simulink library "Energy_converter_Electrical_to_Mechanical"  (R2016a)
settings: Solver=ode1  StartTime=0.0  StopTime=Inf  FixedStep=0.001  RelTol=1e-3
undefined symbols (not defined in the file): API1dcac_efficiency, API2dcac_efficiency, API3dcac_efficiency, aux_power_state, AWR_InvStError, dat, DiscIntNeverNeededParam, EDCU_p_RefTqeMOT, emot_AcCmprFront_inertia, emot_AcCmprFront_nTab_3rdD, emot_AcCmprFront_pwrAC, emot_AcCmprFront_Tau, emot_AcCmprFront_trqTab_2ndD, emot_AcCmprFront_vltTab_1stD, emot_AcCmprRear_inertia, emot_AcCmprRear_nTab_3rdD, emot_AcCmprRear_pwrAC, emot_AcCmprRear_Tau, emot_AcCmprRear_trqTab_2ndD, emot_AcCmprRear_vltTab_1stD, emot_AirCmpr_inertia, emot_AirCmpr_nTab_3rdD, emot_AirCmpr_pwrAC, emot_AirCmpr_Tau, emot_AirCmpr_trqTab_2ndD, emot_AirCmpr_vltTab_1stD, emot_aircomp_power, emot_Cth_rotor, emot_Cth_stator, emot_dtrqEmotNeg, emot_dtrqEmotPtv, emot_inv_pwracTab_1st, emot_inv_pwrDC, emot_inv_pwrLoss, emot_inv_VrmsTab_2nd, emot_j, emot_mot_pwrLoss, emot_nTab_1stD, emot_pwrEtaTab_nRow, emot_pwrEtaTab_pwrTab, emot_pwrEtaTab_trqClm, emot_Rth_rotor_oil, emot_Rth_stator_oil, emot_Rth_stator_rotor, emot_tractiongroup, emot_Trotor_init, emot_trqMaxRow, emot_trqMinRow, emot_Tstator_init, emot_vltTab_3rdD, FirstDrivenAxleNoOfEmot, inv_Cth_cooling_plate, inv_Cth_diode, inv_Cth_IGBT, inv_n_IGBT_per_Switch, inv_Rth_cooling_plate_coolant, inv_Rth_PS_cooling_plate, inv_Tplate_init, inv_Tpowerstack_init, midAxleNoOfEmot ... (+6)
libraries: Electrical_converter x12, Energy_converter_Electrical_to_Mechanical x12, simulink x7
(part 3 of 8)

== system Energy_converter_Electrical_to_Mechanical/Emot AC Compressor Front ==
  hvs_emot_AcCompressorFront_torque : Inport
  hvs_DcLink_voltage_API1 : Inport  Port=2
  hvsAux_InverterAcCompressorFront_torque_Rq : Inport  Port=3
  hvsaux_EmotAcCompressorFront_Voltage_Rq : Inport  Port=4
  Avoid_Div_by_zero : Subsystem
  Constant1 : Constant  Value=0
  Constant2 : Constant  Value=0
  Constant5 : Constant  Value=emot_AcCmprFront_inertia
  Discrete Filter : DiscreteFilter  Numerator=[emot_AcCmprFront_Tau emot_AcCmprFront_Tau]  Denominator=[0.1+emot_AcCmprFront_Tau emot_AcCmprFront_Tau-0.1]
  Discrete-Time Integrator : DiscreteIntegrator  SampleTime=-1  ICPrevOutput=DiscIntNeverNeededParam  ICPrevScaledInput=DiscIntNeverNeededParam
  Gain1 : Gain
      settings: AttributesFormatString=%<Description>
  Gain2 : Gain  SampleTime=K
      mask init:
      | K = str2num(get_param(bdroot,'FixedStep'));
  Gain3 : Gain  Gain=30/pi
      settings: AttributesFormatString=%<Description>
  Product1 : Product  Inputs=*/  RndMeth=Zero
  Product2 : Product  Inputs=**  RndMeth=Zero
  Rate Transition : RateTransition
  Rate Transition1 : RateTransition
  Saturation : Saturate  UpperLimit=Inf  LowerLimit=0
  Subtract : Sum  Inputs=+-
  Subtract1 : Sum  Inputs=+-
  Switch : Switch  Criteria=u2 > Threshold
  W_to_kW : Gain  Gain=1/1000
      settings: AttributesFormatString=%<Description>
  efficiency : Gain  Gain=1/API3dcac_efficiency
      settings: AttributesFormatString=%<Description>
  motor mode : Lookup_n-D  NumberOfTableDimensions=3  BreakpointsForDimension1=emot_AcCmprFront_vltTab_1stD  BreakpointsForDimension2=emot_AcCmprFront_trqTab_2ndD  BreakpointsForDimension3=emot_AcCmprFront_nTab_3rdD  Table=emot_AcCmprFront_pwrAC  ExtrapMethod=Clip  UseLastTableValue=on  InputSameDT=on
  hvs_emot_AirCondFrontHV_angAcc : Outport
  hvs_emot_AirCondFrontHV_angPos : Outport  Port=2
  hvs_emot_AirCondFrontHV_angVel : Outport  Port=3
  hvs_inverterAcCompressor_wasteHeat_power : Outport  Port=4
  hvs_InverterAcCompressorFront_hvCurrent : Outport  Port=5
  hvs_InverterAcCompressorFront_hvVoltage : Outport  Port=6
  hvs_emot_AcCompressorFront_nEmot : Outport  Port=7
  wires:
  W_to_kW/1 -> hvs_inverterAcCompressor_wasteHeat_power/1
  Gain2/1 -> Switch/2, motor mode/2, Subtract/1
  Subtract1/1 -> W_to_kW/1
  efficiency/1 -> Product2/1, Subtract1/1
  Switch/1 -> efficiency/1, Subtract1/2  "phys_current_A"
  Product2/1 -> hvs_InverterAcCompressorFront_hvCurrent/1
  Avoid_Div_by_zero/1(1/U) -> Product2/2
  hvs_DcLink_voltage_API1/1 -> Gain1/1, Avoid_Div_by_zero/1(U)
  Gain1/1 -> hvs_InverterAcCompressorFront_hvVoltage/1
  Constant1/1 -> Switch/3
  Constant2/1 -> hvs_emot_AirCondFrontHV_angPos/1
  hvsAux_InverterAcCompressorFront_torque_Rq/1 -> Discrete Filter/1
  hvsaux_EmotAcCompressorFront_Voltage_Rq/1 -> motor mode/1
  motor mode/1 -> Switch/1  "ElecMac_ElecPwr_W"
  Discrete Filter/1 -> Gain2/1
  hvs_emot_AcCompressorFront_torque/1 -> Subtract/2
  Subtract/1 -> Product1/1
  Constant5/1 -> Product1/2  "phys_inertia_kgm2"
  Product1/1 -> hvs_emot_AirCondFrontHV_angAcc/1, Rate Transition/1
  Discrete-Time Integrator/1 -> Saturation/1
  Saturation/1 -> hvs_emot_AirCondFrontHV_angVel/1, Gain3/1
  Rate Transition/1 -> Discrete-Time Integrator/1
  [angVel] -> Rate Transition1/1
  Rate Transition1/1 -> motor mode/3
  Gain3/1 -> hvs_emot_AcCompressorFront_nEmot/1, [angVel]

== system Energy_converter_Electrical_to_Mechanical/Emot AC Compressor Rear ==
  hvs_emot_AcCompressorRear_torque : Inport
  hvs_DcLink_voltage_API3 : Inport  Port=2
  hvsAux_InverterAcCompressorRear_torque_Rq : Inport  Port=3
  hvsaux_EmotAcCompressorRear_Voltage_Rq : Inport  Port=4
  Avoid_Div_by_zero : Subsystem
  Constant1 : Constant  Value=0
  Constant2 : Constant  Value=0
  Constant5 : Constant  Value=emot_AcCmprRear_inertia
  Discrete Filter : DiscreteFilter  Numerator=[emot_AcCmprRear_Tau emot_AcCmprRear_Tau]  Denominator=[0.1+emot_AcCmprRear_Tau emot_AcCmprRear_Tau-0.1]
  Discrete-Time Integrator : DiscreteIntegrator  SampleTime=-1  ICPrevOutput=DiscIntNeverNeededParam  ICPrevScaledInput=DiscIntNeverNeededParam
  Gain1 : Gain
      settings: AttributesFormatString=%<Description>
  Gain2 : Gain  SampleTime=K
      mask init:
      | K = str2num(get_param(bdroot,'FixedStep'));
  Gain3 : Gain  Gain=30/pi
      settings: AttributesFormatString=%<Description>
  Product1 : Product  Inputs=*/  RndMeth=Zero
  Product2 : Product  Inputs=**  RndMeth=Zero
  Rate Transition1 : RateTransition
  Rate Transition2 : RateTransition
  Saturation : Saturate  UpperLimit=Inf  LowerLimit=0
  Subtract : Sum  Inputs=+-
  Subtract1 : Sum  Inputs=+-
  Switch : Switch  Criteria=u2 > Threshold
  W_to_kW : Gain  Gain=1/1000
      settings: AttributesFormatString=%<Description>
  efficiency : Gain  Gain=1/API1dcac_efficiency
      settings: AttributesFormatString=%<Description>
  motor mode : Lookup_n-D  NumberOfTableDimensions=3  BreakpointsForDimension1=emot_AcCmprRear_vltTab_1stD  BreakpointsForDimension2=emot_AcCmprRear_trqTab_2ndD  BreakpointsForDimension3=emot_AcCmprRear_nTab_3rdD  Table=emot_AcCmprRear_pwrAC  ExtrapMethod=Clip  UseLastTableValue=on  InputSameDT=on
  hvs_emot_AirCondRearHV_angAcc : Outport
  hvs_emot_AirCondRearHV_angPos : Outport  Port=2
  hvs_emot_AirCondRearHV_angVel : Outport  Port=3
  hvs_inverterAcCompressorRear_wasteHeat_power : Outport  Port=4
  hvs_InverterAcCompressorRear_hvCurrent : Outport  Port=5
  hvs_InverterAcCompressorRear_hvVoltage : Outport  Port=6
  hvs_InverterAcCompressorRear_nEmot : Outport  Port=7
  wires:
  W_to_kW/1 -> hvs_inverterAcCompressorRear_wasteHeat_power/1
  Gain2/1 -> Subtract/1, Switch/2, motor mode/2
  Subtract1/1 -> W_to_kW/1
  efficiency/1 -> Subtract1/1, Product2/1
  Switch/1 -> efficiency/1, Subtract1/2  "phys_current_A"
  Avoid_Div_by_zero/1(1/U) -> Product2/2
  Product2/1 -> hvs_InverterAcCompressorRear_hvCurrent/1
  Gain1/1 -> hvs_InverterAcCompressorRear_hvVoltage/1
  hvs_DcLink_voltage_API3/1 -> Gain1/1, Avoid_Div_by_zero/1(U)
  Constant1/1 -> Switch/3
  Saturation/1 -> hvs_emot_AirCondRearHV_angVel/1, Gain3/1
  Discrete-Time Integrator/1 -> Saturation/1
  Product1/1 -> Rate Transition1/1, hvs_emot_AirCondRearHV_angAcc/1
  Constant5/1 -> Product1/2  "phys_inertia_kgm2"
  Subtract/1 -> Product1/1
  hvs_emot_AcCompressorRear_torque/1 -> Subtract/2
  Discrete Filter/1 -> Gain2/1
  motor mode/1 -> Switch/1  "ElecMac_ElecPwr_W"
  hvsaux_EmotAcCompressorRear_Voltage_Rq/1 -> motor mode/1
  hvsAux_InverterAcCompressorRear_torque_Rq/1 -> Discrete Filter/1
  Constant2/1 -> hvs_emot_AirCondRearHV_angPos/1
  Rate Transition1/1 -> Discrete-Time Integrator/1
  [angVel] -> Rate Transition2/1
  Rate Transition2/1 -> motor mode/3
  Gain3/1 -> [angVel], hvs_InverterAcCompressorRear_nEmot/1

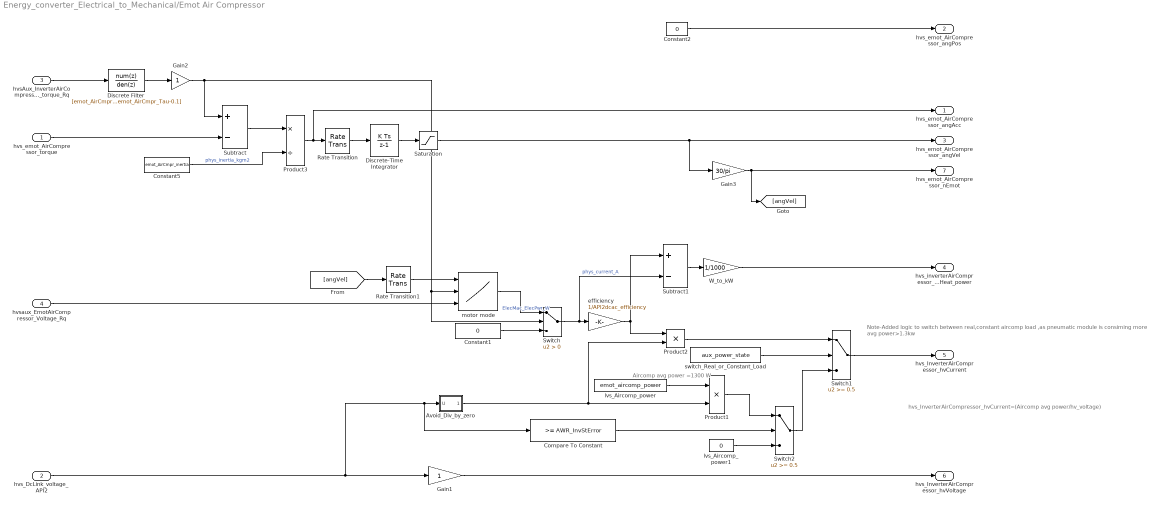
== system Energy_converter_Electrical_to_Mechanical/Emot Air Compressor ==
  note: Note-Added logic to switch between real,constant aircomp load ,as pneumatic module is consiming more avg power>1.3kw
  note: hvs_InverterAirCompressor_hvCurrent=(Aircomp avg power/hv_voltage)
  note: Aircomp avg power =1300 W
  hvs_emot_AirCompressor_torque : Inport
  hvs_DcLink_voltage_API2 : Inport  Port=2
  hvsAux_InverterAirCompressor_torque_Rq : Inport  Port=3
  hvsaux_EmotAirCompressor_Voltage_Rq : Inport  Port=4
  Avoid_Div_by_zero : Subsystem
  Compare To Constant : simulink/Logic and Bit Operations/Compare To Constant  relop=>=  const=AWR_InvStError  OutDataTypeStr=boolean
  Constant1 : Constant  Value=0
  Constant2 : Constant  Value=0
  Constant5 : Constant  Value=emot_AirCmpr_inertia
  Discrete Filter : DiscreteFilter  Numerator=[emot_AirCmpr_Tau emot_AirCmpr_Tau]  Denominator=[0.1+emot_AirCmpr_Tau emot_AirCmpr_Tau-0.1]
  Discrete-Time Integrator : DiscreteIntegrator  SampleTime=-1  ICPrevOutput=DiscIntNeverNeededParam  ICPrevScaledInput=DiscIntNeverNeededParam
  Gain1 : Gain
      settings: AttributesFormatString=%<Description>
  Gain2 : Gain  SampleTime=K
      mask init:
      | K = str2num(get_param(bdroot,'FixedStep'));
  Gain3 : Gain  Gain=30/pi
      settings: AttributesFormatString=%<Description>
  Product1 : Product  Inputs=**  RndMeth=Zero
  Product2 : Product  Inputs=**  RndMeth=Zero
  Product3 : Product  Inputs=*/  RndMeth=Zero
  Rate Transition : RateTransition
  Rate Transition1 : RateTransition
  Saturation : Saturate  UpperLimit=inf  LowerLimit=0
  Subtract : Sum  Inputs=+-
  Subtract1 : Sum  Inputs=+-
  Switch : Switch  Criteria=u2 > Threshold
  Switch1 : Switch  Threshold=0.5
  Switch2 : Switch  Threshold=0.5
  W_to_kW : Gain  Gain=1/1000
      settings: AttributesFormatString=%<Description>
  efficiency : Gain  Gain=1/API2dcac_efficiency
      settings: AttributesFormatString=%<Description>
  lvs_Aircomp_power : Constant  Value=emot_aircomp_power
  lvs_Aircomp_power1 : Constant  Value=0
  motor mode : Lookup_n-D  NumberOfTableDimensions=3  BreakpointsForDimension1=emot_AirCmpr_nTab_3rdD  BreakpointsForDimension2=emot_AirCmpr_trqTab_2ndD  BreakpointsForDimension3=emot_AirCmpr_vltTab_1stD  Table=emot_AirCmpr_pwrAC  ExtrapMethod=Clip  UseLastTableValue=on  InputSameDT=on
  switch_Real_or_Constant_Load : Constant  Value=aux_power_state
  hvs_emot_AirCompressor_angAcc : Outport
  hvs_emot_AirCompressor_angPos : Outport  Port=2
  hvs_emot_AirCompressor_angVel : Outport  Port=3
  hvs_inverterAirCompressor_wasteHeat_power : Outport  Port=4
  hvs_InverterAirCompressor_hvCurrent : Outport  Port=5
  hvs_InverterAirCompressor_hvVoltage : Outport  Port=6
  hvs_emot_AirCompressor_nEmot : Outport  Port=7
  wires:
  Switch2/1 -> Switch1/3
  Product1/1 -> Switch2/1
  Compare To Constant/1 -> Switch2/2
  lvs_Aircomp_power/1 -> Product1/1
  lvs_Aircomp_power1/1 -> Switch2/3
  hvs_DcLink_voltage_API2/1 -> Gain1/1, Avoid_Div_by_zero/1(U), Compare To Constant/1
  switch_Real_or_Constant_Load/1 -> Switch1/2
  Product2/1 -> Switch1/1
  Gain3/1 -> hvs_emot_AirCompressor_nEmot/1, [angVel]
  W_to_kW/1 -> hvs_inverterAirCompressor_wasteHeat_power/1
  Gain2/1 -> Subtract/1, Switch/2, motor mode/2
  Subtract1/1 -> W_to_kW/1
  efficiency/1 -> Product2/1, Subtract1/1
  Constant1/1 -> Switch/3
  Avoid_Div_by_zero/1(1/U) -> Product1/2, Product2/2
  Switch/1 -> efficiency/1, Subtract1/2  "phys_current_A"
  Gain1/1 -> hvs_InverterAirCompressor_hvVoltage/1
  hvsaux_EmotAirCompressor_Voltage_Rq/1 -> motor mode/3
  Saturation/1 -> hvs_emot_AirCompressor_angVel/1, Gain3/1
  Discrete-Time Integrator/1 -> Saturation/1
  Product3/1 -> Rate Transition/1, hvs_emot_AirCompressor_angAcc/1
  Constant5/1 -> Product3/2  "phys_inertia_kgm2"
  Subtract/1 -> Product3/1
  hvs_emot_AirCompressor_torque/1 -> Subtract/2
  Discrete Filter/1 -> Gain2/1
  motor mode/1 -> Switch/1  "ElecMac_ElecPwr_W"
  hvsAux_InverterAirCompressor_torque_Rq/1 -> Discrete Filter/1
  Constant2/1 -> hvs_emot_AirCompressor_angPos/1
  Rate Transition/1 -> Discrete-Time Integrator/1
  [angVel] -> Rate Transition1/1
  Rate Transition1/1 -> motor mode/1
  Switch1/1 -> hvs_InverterAirCompressor_hvCurrent/1

== system Energy_converter_Electrical_to_Mechanical/GTR_Electric_machine ==
  ElecMac_nReq_radps : Inport
  ElecMac_flgReqSwitch_B : Inport  Port=2
  ElecMac_tqReq_Nm : Inport  Port=3
  ElecMac_flowActCooling_kgps : Inport  Port=4
  el in [V] : Inport  Port=5
  mech fb in [rad/s] : Inport  Port=6
  Bus Creator : BusCreator  Inputs=2
  Bus Creator1 : BusCreator  Inputs=1
  Bus Creator2 : BusCreator  Inputs=5
  Bus Selector1 : BusSelector  OutputSignals=phys_voltage_V
  Bus Selector2 : BusSelector  OutputSignals=phys_speed_radps
  Bus Selector3 : BusSelector  OutputSignals=torque,ElecMac_flowActCooling_kgps
  Constant1 : Constant  Value=dat.inertia.value
  Gain{1..3,6} (4 alike) : Gain
  Product : Product  Inputs=/*  RndMeth=Zero
  Product1 : Product  Inputs=**  RndMeth=Zero
  Sum : Sum  Inputs=+-
  Switch : Switch
  Thermal : Subsystem
  Transfer Fcn1 : TransferFcn  Denominator=[dat.timeconstant.value 1]
  generator mode : Lookup_n-D  NumberOfTableDimensions=3  BreakpointsForDimension1=dat.elecpowmap.generator.voltage.vec  BreakpointsForDimension2=dat.elecpowmap.generator.torque.vec  BreakpointsForDimension3=dat.elecpowmap.generator.speed.vec  Table=dat.elecpowmap.generator.elecpow.map  ExtrapMethod=Clip  UseLastTableValue=on  InputSameDT=on
  local controller : Subsystem
  motor mode : Lookup_n-D  NumberOfTableDimensions=3  BreakpointsForDimension1=dat.elecpowmap.motor.voltage.vec  BreakpointsForDimension2=dat.elecpowmap.motor.torque.vec  BreakpointsForDimension3=dat.elecpowmap.motor.speed.vec  Table=dat.elecpowmap.motor.elecpow.map  ExtrapMethod=Clip  UseLastTableValue=on  InputSameDT=on
  mech out [Nm] : Outport
  el fb out [A] : Outport  Port=2
  Electric_speed_radps : Outport  Port=3
  wires:
  Sum/1 -> Thermal/1(Total power loss)
  Product1/1 -> Sum/2
  Thermal/1(Machine temperature[K]) -> Bus Creator2/4  "ElecMac_tAct_K"
  Gain6/1 -> Bus Creator/1  "phys_torque_Nm"
  Gain2/1 -> Bus Creator2/1  "ElecMac_tqAct_Nm"
  Gain1/1 -> Bus Creator2/2  "ElecMac_nAct_radps"
  Gain3/1 -> Bus Creator2/3  "ElecMac_iAct_A"
  Product/1 -> Gain3/1, Bus Creator1/1  "phys_current_A"
  Bus Selector3/1 -> Transfer Fcn1/1  "<torque>"
  Constant1/1 -> Bus Creator/2  "phys_inertia_kgm2"
  Bus Creator2/1 -> local controller/5(sensor in)
  Bus Selector2/1 -> Gain1/1, Product1/2, generator mode/3, motor mode/3  "<phys_speed_radps>"
  local controller/2(ctrl out) -> Bus Selector3/1
  mech fb in [rad/s]/1 -> Bus Selector2/1
  el in [V]/1 -> Bus Selector1/1
  Bus Creator/1 -> mech out [Nm]/1
  Bus Creator1/1 -> el fb out [A]/1
  motor mode/1 -> Switch/1  "ElecMac_ElecPwr_W"
  generator mode/1 -> Switch/3
  Switch/1 -> Product/2, Sum/1
  Bus Selector1/1 -> Product/1, motor mode/1, generator mode/1  "<phys_voltage_V>"
  Transfer Fcn1/1 -> Gain2/1, Gain6/1, Product1/1, generator mode/2, Switch/2, motor mode/2
  Bus Selector3/2 -> Thermal/2(Massflow cooling fluid)  "<ElecMac_flowActCooling_kgps>"
  Thermal/2(Fluid outlet temperature[K]) -> Bus Creator2/5  "ElecMac_tActCoolingOut_K"
  local controller/1(Electric_speed_radps) -> Electric_speed_radps/1
  ElecMac_nReq_radps/1 -> local controller/1(ElecMac_nReq_radps)
  ElecMac_flgReqSwitch_B/1 -> local controller/2(ElecMac_flgReqSwitch_B)
  ElecMac_tqReq_Nm/1 -> local controller/3(ElecMac_tqReq_Nm)
  ElecMac_flowActCooling_kgps/1 -> local controller/4(ElecMac_flowActCooling_kgps)

== system Energy_converter_Electrical_to_Mechanical/e-Motor ==
  nGbxEMIn : Inport
  voltBatHV : Inport  Port=2
  trqEmotDesPhy : Inport  Port=3
  emot_CMD : Inport  Port=4
  drvEmotOil_Temperature : Inport  Port=5
  drvInverter_Coolant_Temperature : Inport  Port=6
  Enable : EnablePort
  Constant2 : Constant  Value=0
  Fahrmotoren : Subsystem
  Gain : Gain  Gain=0.4
  Gain1 : Gain  Gain=0.6
  Switch : Switch  Threshold=0.5
  Thermic_Model_Inverter : Subsystem
  Thermic_Model_PMSM_slot2 : Subsystem
  Umrichter mit trq-Regler : Subsystem
  Unit Delay : UnitDelay  SampleTime=-1
  Unit Delay1 : UnitDelay  InitialCondition=emot_Tstator_init  SampleTime=-1
  Unit Delay2 : UnitDelay  InitialCondition=emot_Trotor_init  SampleTime=-1
  Unit Delay4 : UnitDelay  InitialCondition=inv_Tpowerstack_init  SampleTime=-1
  Unit Delay5 : UnitDelay  InitialCondition=inv_Tplate_init  SampleTime=-1
  updatePortNames : Subsystem
      settings: OpenFcn=std_PortNameFromSignal('Depth',2);
      mask Display: disp('updatePortNames')
  pwrEmotPhy : Outport
  Inv_Ploss : Outport  Port=2
  mot_Ploss : Outport  Port=3
  trqEmotPhy : Outport  Port=4
  trqEmotMax : Outport  Port=5
  drvEmot_wasteHeat_power : Outport  Port=6
  drvEmot_T_Stator : Outport  Port=7
  driveInverter_wasteHeat_power : Outport  Port=8
  driveInverter_T_Coolplate : Outport  Port=9
  wires:
  Thermic_Model_PMSM_slot2/3(T_Rotor_new) -> Unit Delay1/1  "drvEmot_T_Rotor"
  Unit Delay1/1 -> Thermic_Model_PMSM_slot2/5(T_Rotor)
  Thermic_Model_PMSM_slot2/2(T_Stator_new) -> drvEmot_T_Stator/1, Unit Delay2/1  "drvEmot_T_Stator"
  Unit Delay2/1 -> Thermic_Model_PMSM_slot2/4(T_Stator)
  Gain/1 -> Thermic_Model_PMSM_slot2/1(P_WasteHeat_Rotor)
  Gain1/1 -> Thermic_Model_PMSM_slot2/2(P_WasteHeat_Stator)
  [mot_Ploss] -> Gain1/1, Gain/1
  drvEmotOil_Temperature/1 -> Thermic_Model_PMSM_slot2/3(T_Oil)
  Thermic_Model_PMSM_slot2/1(HeatFlow_eMotor_Oil) -> drvEmot_wasteHeat_power/1  "drvEmot_wasteHeat_power"
  [Inv_Ploss] -> Thermic_Model_Inverter/1(P_WasteHeat_Powerstack)
  Thermic_Model_Inverter/3(T_Plate_new) -> driveInverter_T_Coolplate/1, Unit Delay4/1  "driveInverter_T_plate"
  Unit Delay4/1 -> Thermic_Model_Inverter/4(T_Plate)
  Thermic_Model_Inverter/2(T_Powerstack_new) -> Unit Delay5/1  "driveInverter_T_PS"
  Unit Delay5/1 -> Thermic_Model_Inverter/3(T_Powerstack)
  Thermic_Model_Inverter/1(P_Coolant) -> driveInverter_wasteHeat_power/1  "driveInverter_wasteHeat_power"
  drvInverter_Coolant_Temperature/1 -> Thermic_Model_Inverter/2(T_Coolant)
  Unit Delay/1 -> Umrichter mit trq-Regler/5(mot_Ploss)
  Constant2/1 -> Switch/3
  [EMD_CMD] -> Switch/2
  Fahrmotoren/1(mot_Ploss) -> Switch/1, Unit Delay/1
  emot_CMD/1 -> Umrichter mit trq-Regler/4(emot_CMD), [EMD_CMD]
  Umrichter mit trq-Regler/10(trqEmotMax) -> trqEmotMax/1  "trqEmotMax"
  Umrichter mit trq-Regler/1(pwrInv_dc) -> pwrEmotPhy/1  "pwrEmotPhy"
  Umrichter mit trq-Regler/2(inv_Ploss) -> [Inv_Ploss], Inv_Ploss/1  "Inv_Ploss"
  Umrichter mit trq-Regler/4(nEmot_f) -> Fahrmotoren/2(nEmot_f)
  Umrichter mit trq-Regler/3(nEmot_k) -> Fahrmotoren/1(nEmot_k)
  Umrichter mit trq-Regler/9(trqEmot_raw) -> trqEmotPhy/1  "trqEmotPhy"
  Umrichter mit trq-Regler/5(trqEmot_k) -> Fahrmotoren/3(trqEmot_k)
  Umrichter mit trq-Regler/6(trqEmot_f) -> Fahrmotoren/4(trqEmot_f)
  Umrichter mit trq-Regler/7(U_DC_k) -> Fahrmotoren/5(U_DC_k)
  Umrichter mit trq-Regler/8(U_DC_f) -> Fahrmotoren/6(U_DC_f)
  Switch/1 -> mot_Ploss/1, [mot_Ploss]  "mot_Ploss"
  nGbxEMIn/1 -> Umrichter mit trq-Regler/3(nEmot)
  voltBatHV/1 -> Umrichter mit trq-Regler/2(U_ZK)
  trqEmotDesPhy/1 -> Umrichter mit trq-Regler/1(trqDes)

== system Energy_converter_Electrical_to_Mechanical/e-Motor_Gen2 ==
  nGbxEMIn : Inport
  voltBatHV : Inport  Port=2
  trqEmotDesPhy : Inport  Port=3
  emot_CMD : Inport  Port=4
  drvEmotOil_Temperature : Inport  Port=5
  drvInverter_Coolant_Temperature : Inport  Port=6
  Enable : EnablePort
  Constant2 : Constant  Value=0
  Fahrmotoren : Subsystem
  Gain : Gain  Gain=0.4
  Gain1 : Gain  Gain=0.6
  Switch : Switch  Threshold=0.5
  Thermic_Model_Inverter : Subsystem
  Thermic_Model_PMSM_slot2 : Subsystem
  Umrichter mit trq-Regler : Subsystem
  Unit Delay : UnitDelay  SampleTime=-1
  Unit Delay1 : UnitDelay  InitialCondition=emot_Tstator_init  SampleTime=-1
  Unit Delay2 : UnitDelay  InitialCondition=emot_Trotor_init  SampleTime=-1
  Unit Delay4 : UnitDelay  InitialCondition=inv_Tpowerstack_init  SampleTime=-1
  Unit Delay5 : UnitDelay  InitialCondition=inv_Tplate_init  SampleTime=-1
  updatePortNames : Subsystem
      settings: OpenFcn=std_PortNameFromSignal('Depth',2);
      mask Display: disp('updatePortNames')
  pwrEmotPhy : Outport
  Inv_Ploss : Outport  Port=2
  mot_Ploss : Outport  Port=3
  trqEmotPhy : Outport  Port=4
  trqEmotMax : Outport  Port=5
  drvEmot_wasteHeat_power : Outport  Port=6
  drvEmot_T_Stator : Outport  Port=7
  driveInverter_wasteHeat_power : Outport  Port=8
  driveInverter_T_Coolplate : Outport  Port=9
  wires:
  Unit Delay/1 -> Umrichter mit trq-Regler/5(mot_Ploss)
  Constant2/1 -> Switch/3
  [EMD_CMD] -> Switch/2
  Fahrmotoren/1(mot_Ploss) -> Unit Delay/1, Switch/1
  emot_CMD/1 -> Umrichter mit trq-Regler/4(emot_CMD), [EMD_CMD]
  Umrichter mit trq-Regler/4(trqEmotMax) -> trqEmotMax/1  "trqEmotMax"
  Umrichter mit trq-Regler/1(pwrInv_dc) -> pwrEmotPhy/1  "pwrEmotPhy"
  Umrichter mit trq-Regler/2(inv_Ploss) -> [Inv_Ploss], Inv_Ploss/1  "Inv_Ploss"
  Umrichter mit trq-Regler/6(nEmot_f) -> Fahrmotoren/2(nEmot_f)
  Umrichter mit trq-Regler/5(nEmot_k) -> Fahrmotoren/1(nEmot_k)
  Umrichter mit trq-Regler/3(trqEmot_raw) -> trqEmotPhy/1  "trqEmotPhy"
  Umrichter mit trq-Regler/7(trqEmot_k) -> Fahrmotoren/3(trqEmot_k)
  Umrichter mit trq-Regler/8(trqEmot_f) -> Fahrmotoren/4(trqEmot_f)
  Umrichter mit trq-Regler/9(U_DC_k) -> Fahrmotoren/5(U_DC_k)
  Umrichter mit trq-Regler/10(U_DC_f) -> Fahrmotoren/6(U_DC_f)
  Switch/1 -> [mot_Ploss], mot_Ploss/1  "mot_Ploss"
  nGbxEMIn/1 -> Umrichter mit trq-Regler/3(nEmot)
  voltBatHV/1 -> Umrichter mit trq-Regler/2(U_ZK)
  trqEmotDesPhy/1 -> Umrichter mit trq-Regler/1(trqDes)
  Thermic_Model_PMSM_slot2/3(T_Rotor_new) -> Unit Delay1/1  "drvEmot_T_Rotor"
  Unit Delay1/1 -> Thermic_Model_PMSM_slot2/5(T_Rotor)
  Thermic_Model_PMSM_slot2/2(T_Stator_new) -> drvEmot_T_Stator/1, Unit Delay2/1  "drvEmot_T_Stator"
  Unit Delay2/1 -> Thermic_Model_PMSM_slot2/4(T_Stator)
  Gain/1 -> Thermic_Model_PMSM_slot2/1(P_WasteHeat_Rotor)
  Gain1/1 -> Thermic_Model_PMSM_slot2/2(P_WasteHeat_Stator)
  [mot_Ploss] -> Gain1/1, Gain/1
  drvEmotOil_Temperature/1 -> Thermic_Model_PMSM_slot2/3(T_Oil)
  Thermic_Model_PMSM_slot2/1(HeatFlow_eMotor_Oil) -> drvEmot_wasteHeat_power/1  "drvEmot_wasteHeat_power"
  [Inv_Ploss] -> Thermic_Model_Inverter/1(P_WasteHeat_Powerstack)
  Thermic_Model_Inverter/3(T_Plate_new) -> driveInverter_T_Coolplate/1, Unit Delay4/1  "driveInverter_T_plate"
  Unit Delay4/1 -> Thermic_Model_Inverter/4(T_Plate)
  Thermic_Model_Inverter/2(T_Powerstack_new) -> Unit Delay5/1  "driveInverter_T_PS"
  Unit Delay5/1 -> Thermic_Model_Inverter/3(T_Powerstack)
  Thermic_Model_Inverter/1(P_Coolant) -> driveInverter_wasteHeat_power/1  "driveInverter_wasteHeat_power"
  drvInverter_Coolant_Temperature/1 -> Thermic_Model_Inverter/2(T_Coolant)

== system Energy_converter_Electrical_to_Mechanical/e-Motor_chy_proposal ==
  note: Orange blocks: to be deleted?
  nGbxEMIn : Inport
  voltBatHV : Inport  Port=2
  trqEmotDesPhy : Inport  Port=3
  ndotGbxEMIn : Inport  Port=4
  Add : Sum
  Constant : Constant  Value=emot_j
      settings: AttributesFormatString=%<Value>
  Constant1 : Constant  Value=1/1.01
  Constant2 : Constant  Value=-650
  Constant3 : Constant  Value=0
  Constant4 : Constant
  Fahrmotoren : Subsystem
  Manual Switch : ManualSwitch  CurrentSetting=0
  Manual Switch1 : ManualSwitch  CurrentSetting=0
  Memory : Memory
  Product : Product  RndMeth=Zero
  Product1 : Product  RndMeth=Zero
  Sum : Sum  Inputs=|+-
  Umrichter mit trq-Regler : Subsystem
  rpm2Radps1 : Gain  Gain=pi/30
  updatePortNames : Subsystem
      settings: OpenFcn=std_PortNameFromSignal('Depth',2);
      mask Display: disp('updatePortNames')
  pwrEmotPhy : Outport
  Inv_Ploss : Outport  Port=2
  mot_Ploss : Outport  Port=3
  trqEmotPhy : Outport  Port=4
  trqEmotMax : Outport  Port=5
  pwrEmotMax : Outport  Port=6
  wires:
  Umrichter mit trq-Regler/11(pwrInvmax) -> pwrEmotMax/1  "pwrEmotMax"
  Umrichter mit trq-Regler/10(trqEmotMax) -> trqEmotMax/1  "trqEmotMax"
  Constant/1 -> Product/2  "jEmotPhy"
  Umrichter mit trq-Regler/1(pwrInv_dc) -> Product1/2  "pwrEmotPhy"
  Sum/1 -> trqEmotPhy/1  "trqEmotPhy"
  Umrichter mit trq-Regler/2(inv_Ploss) -> Inv_Ploss/1  "Inv_Ploss"
  Umrichter mit trq-Regler/4(nEmot_f) -> Fahrmotoren/2(nEmot_f)
  Umrichter mit trq-Regler/3(nEmot_k) -> Fahrmotoren/1(nEmot_k)
  rpm2Radps1/1 -> Memory/1
  Memory/1 -> Product/1
  Umrichter mit trq-Regler/9(trqEmot_raw) -> Sum/1  "trqEmotPhy"
  Product/1 -> Sum/2
  Umrichter mit trq-Regler/5(trqEmot_k) -> Fahrmotoren/3(trqEmot_k)
  Umrichter mit trq-Regler/6(trqEmot_f) -> Fahrmotoren/4(trqEmot_f)
  Umrichter mit trq-Regler/7(U_DC_k) -> Fahrmotoren/5(U_DC_k)
  Umrichter mit trq-Regler/8(U_DC_f) -> Fahrmotoren/6(U_DC_f)
  Fahrmotoren/1(mot_Ploss) -> mot_Ploss/1  "mot_Ploss"
  Product1/1 -> Add/2  "pwrEmotPhy"
  Add/1 -> pwrEmotPhy/1  "pwrEmotPhy"
  Constant1/1 -> Manual Switch/1
  Constant4/1 -> Manual Switch/2
  Manual Switch/1 -> Product1/1
  Constant2/1 -> Manual Switch1/1
  Constant3/1 -> Manual Switch1/2
  Manual Switch1/1 -> Add/1
  ndotGbxEMIn/1 -> rpm2Radps1/1
  nGbxEMIn/1 -> Umrichter mit trq-Regler/3(nEmot)
  voltBatHV/1 -> Umrichter mit trq-Regler/2(U_ZK)
  trqEmotDesPhy/1 -> Umrichter mit trq-Regler/1(trqDes)

== system Energy_converter_Electrical_to_Mechanical/AWR_DriveEmot/AWR 1 TX ==
  IN_EMD1_ACT_DcLinkVoltage : Inport
  IN_EMD1_ACT_DigitalInput1 : Inport  Port=2
  IN_EMD1_ACT_MaximumAvailableTorque : Inport  Port=3
  IN_EMD1_ACT_DcLinkPower : Inport  Port=4
  IN_EMD1_ACT_MotorSpeed : Inport  Port=5
  IN_EMD1_ACT_Torque : Inport  Port=6
  IN_EMD1_ACT_InverterState : Inport  Port=7
  IN_EMD1_ACT_ReferenceTorqueLimited : Inport  Port=8
  IN_EMD1_ACT_MaxJunctionTemperature : Inport  Port=9
  IN_EMD1_ACT_MotorTemperature : Inport  Port=10
  IN_EMD1_ACT_InverterLosses : Inport  Port=11
  IN_EMD1_ACT_MotorLosses : Inport  Port=12
  Constant3 : Constant  Value=RefTqeMOT
  Constant39 : Constant  Value=RefTqeMOT
  Constant5 : Constant  Value=RefTqeMOT
  Nm_to_percent : Subsystem
  Nm_to_percent1 : Subsystem
  Nm_to_percent2 : Subsystem
  hvs_EMD1_ACT_DigitalInput1 : Outport
  hvs_EMD1_ACT_InverterState : Outport  Port=2
  hvs_EMD1_ACT_MaxAvailableTorque : Outport  Port=3
  hvs_EMD1_ACT_ReferenceTorqueLim : Outport  Port=4
  hvs_EMD1_ACT_Torque : Outport  Port=5
  hvs_EMD1_ACT_DcLinkPower : Outport  Port=6
  hvs_EMD1_ACT_MotorSpeed : Outport  Port=7
  hvs_EMD1_ACT_DcLinkVoltage : Outport  Port=8
  hvs_EMD1_ACT_MaxJunctionTemp : Outport  Port=9
  hvs_EMD1_ACT_MotorTemperature : Outport  Port=10
  hvs_EMD1_ACT_InverterLosses : Outport  Port=11
  hvs_EMD1_ACT_MotorLosses : Outport  Port=12
  wires:
  IN_EMD1_ACT_MotorLosses/1 -> hvs_EMD1_ACT_MotorLosses/1  "hvs_EMD1_ACT_MotorLosses"
  IN_EMD1_ACT_InverterLosses/1 -> hvs_EMD1_ACT_InverterLosses/1  "hvs_EMD1_ACT_InverterLosses"
  Constant39/1 -> Nm_to_percent2/2(Reference_Torque)
  Nm_to_percent2/1(Torque_Percentage) -> hvs_EMD1_ACT_Torque/1  "hvs_EMD1_ACT_Torque"
  Constant3/1 -> Nm_to_percent/2(Reference_Torque)
  IN_EMD1_ACT_MaximumAvailableTorque/1 -> Nm_to_percent/1(Nm_Torque)  "EMD1_ACT_MaximumAvailableTorque"
  IN_EMD1_ACT_DigitalInput1/1 -> hvs_EMD1_ACT_DigitalInput1/1  "hvs_EMD1_ACT_DigitalInput1"
  IN_EMD1_ACT_MotorTemperature/1 -> hvs_EMD1_ACT_MotorTemperature/1  "hvs_EMD1_ACT_MotorTemperature"
  IN_EMD1_ACT_MaxJunctionTemperature/1 -> hvs_EMD1_ACT_MaxJunctionTemp/1  "hvs_EMD1_ACT_MaxJunctionTemp"
  IN_EMD1_ACT_Torque/1 -> Nm_to_percent2/1(Nm_Torque)
  IN_EMD1_ACT_MotorSpeed/1 -> hvs_EMD1_ACT_MotorSpeed/1  "hvs_EMD1_ACT_MotorSpeed"
  Nm_to_percent1/1(Torque_Percentage) -> hvs_EMD1_ACT_ReferenceTorqueLim/1  "hvs_EMD1_ACT_ReferenceTorqueLim"
  Nm_to_percent/1(Torque_Percentage) -> hvs_EMD1_ACT_MaxAvailableTorque/1  "hvs_EMD1_ACT_MaxAvailableTorque"
  IN_EMD1_ACT_DcLinkVoltage/1 -> hvs_EMD1_ACT_DcLinkVoltage/1  "hvs_EMD1_ACT_DcLinkVoltage"
  IN_EMD1_ACT_DcLinkPower/1 -> hvs_EMD1_ACT_DcLinkPower/1  "hvs_EMD1_ACT_DcLinkPower"
  IN_EMD1_ACT_InverterState/1 -> hvs_EMD1_ACT_InverterState/1  "hvs_EMD1_ACT_InverterState"
  IN_EMD1_ACT_ReferenceTorqueLimited/1 -> Nm_to_percent1/1(Nm_Torque)  "EMD1_ACT_ReferenceTorqueLimited"
  Constant5/1 -> Nm_to_percent1/2(Reference_Torque)

== system Energy_converter_Electrical_to_Mechanical/AWR_DriveEmot/AWR 2 TX ==
  IN_EMD2_ACT_DcLinkVoltage : Inport
  IN_EMD2_ACT_DigitalInput1 : Inport  Port=2
  IN_EMD2_ACT_MaximumAvailableTorque : Inport  Port=3
  IN_EMD2_ACT_DcLinkPower : Inport  Port=4
  IN_EMD2_ACT_MotorSpeed : Inport  Port=5
  IN_EMD2_ACT_Torque : Inport  Port=6
  IN_EMD2_ACT_InverterState : Inport  Port=7
  IN_EMD2_ACT_ReferenceTorqueLimited : Inport  Port=8
  IN_EMD2_ACT_MaxJunctionTemperature : Inport  Port=9
  IN_EMD2_ACT_MotorTemperature : Inport  Port=10
  IN_EMD2_ACT_InverterLosses : Inport  Port=11
  IN_EMD2_ACT_MotorLosses : Inport  Port=12
  Constant3 : Constant  Value=RefTqeMOT
  Constant39 : Constant  Value=RefTqeMOT
  Constant5 : Constant  Value=RefTqeMOT
  Nm_to_percent : Subsystem
  Nm_to_percent1 : Subsystem
  Nm_to_percent2 : Subsystem
  hvs_EMD2_ACT_DigitalInput1 : Outport
  hvs_EMD2_ACT_InverterState : Outport  Port=2
  hvs_EMD2_ACT_MaxAvailableTorque : Outport  Port=3
  hvs_EMD2_ACT_ReferenceTorqueLim : Outport  Port=4
  hvs_EMD2_ACT_Torque : Outport  Port=5
  hvs_EMD2_ACT_DcLinkPower : Outport  Port=6
  hvs_EMD2_ACT_MotorSpeed : Outport  Port=7
  hvs_EMD2_ACT_DcLinkVoltage : Outport  Port=8
  hvs_EMD2_ACT_MaxJunctionTemp : Outport  Port=9
  hvs_EMD2_ACT_MotorTemperature : Outport  Port=10
  hvs_EMD2_ACT_InverterLosses : Outport  Port=11
  hvs_EMD2_ACT_MotorLosses : Outport  Port=12
  wires:
  IN_EMD2_ACT_MotorLosses/1 -> hvs_EMD2_ACT_MotorLosses/1  "hvs_EMD2_ACT_MotorLosses"
  IN_EMD2_ACT_InverterLosses/1 -> hvs_EMD2_ACT_InverterLosses/1  "hvs_EMD2_ACT_InverterLosses"
  Constant39/1 -> Nm_to_percent2/2(Reference_Torque)
  Nm_to_percent2/1(Torque_Percentage) -> hvs_EMD2_ACT_Torque/1  "hvs_EMD2_ACT_Torque"
  Constant3/1 -> Nm_to_percent/2(Reference_Torque)
  IN_EMD2_ACT_MaximumAvailableTorque/1 -> Nm_to_percent/1(Nm_Torque)  "EMD1_ACT_MaximumAvailableTorque"
  IN_EMD2_ACT_DigitalInput1/1 -> hvs_EMD2_ACT_DigitalInput1/1  "hvs_EMD2_ACT_DigitalInput1"
  IN_EMD2_ACT_MotorTemperature/1 -> hvs_EMD2_ACT_MotorTemperature/1  "hvs_EMD2_ACT_MotorTemperature"
  IN_EMD2_ACT_MaxJunctionTemperature/1 -> hvs_EMD2_ACT_MaxJunctionTemp/1  "hvs_EMD2_ACT_MaxJunctionTemp"
  IN_EMD2_ACT_Torque/1 -> Nm_to_percent2/1(Nm_Torque)
  IN_EMD2_ACT_MotorSpeed/1 -> hvs_EMD2_ACT_MotorSpeed/1  "hvs_EMD2_ACT_MotorSpeed"
  Nm_to_percent1/1(Torque_Percentage) -> hvs_EMD2_ACT_ReferenceTorqueLim/1  "hvs_EMD2_ACT_ReferenceTorqueLim"
  Nm_to_percent/1(Torque_Percentage) -> hvs_EMD2_ACT_MaxAvailableTorque/1  "hvs_EMD2_ACT_MaxAvailableTorque"
  IN_EMD2_ACT_DcLinkVoltage/1 -> hvs_EMD2_ACT_DcLinkVoltage/1  "hvs_EMD2_ACT_DcLinkVoltage"
  IN_EMD2_ACT_DcLinkPower/1 -> hvs_EMD2_ACT_DcLinkPower/1  "hvs_EMD2_ACT_DcLinkPower"
  IN_EMD2_ACT_InverterState/1 -> hvs_EMD2_ACT_InverterState/1  "hvs_EMD2_ACT_InverterState"
  IN_EMD2_ACT_ReferenceTorqueLimited/1 -> Nm_to_percent1/1(Nm_Torque)  "EMD1_ACT_ReferenceTorqueLimited"
  Constant5/1 -> Nm_to_percent1/2(Reference_Torque)

== system Energy_converter_Electrical_to_Mechanical/AWR_DriveEmot/AWR 3 TX ==
  IN_EMD3_ACT_DcLinkVoltage : Inport
  IN_EMD3_ACT_DigitalInput1 : Inport  Port=2
  IN_EMD3_ACT_MaximumAvailableTorque : Inport  Port=3
  IN_EMD3_ACT_DcLinkPower : Inport  Port=4
  IN_EMD3_ACT_MotorSpeed : Inport  Port=5
  IN_EMD3_ACT_Torque : Inport  Port=6
  IN_EMD3_ACT_InverterState : Inport  Port=7
  IN_EMD3_ACT_ReferenceTorqueLimited : Inport  Port=8
  IN_EMD3_ACT_MaxJunctionTemperature : Inport  Port=9
  IN_EMD3_ACT_MotorTemperature : Inport  Port=10
  IN_EMD3_ACT_InverterLosses : Inport  Port=11
  IN_EMD3_ACT_MotorLosses : Inport  Port=12
  Constant3 : Constant  Value=RefTqeMOT
  Constant39 : Constant  Value=RefTqeMOT
  Constant5 : Constant  Value=RefTqeMOT
  Nm_to_percent : Subsystem
  Nm_to_percent1 : Subsystem
  Nm_to_percent2 : Subsystem
  hvs_EMD3_ACT_DigitalInput1 : Outport
  hvs_EMD3_ACT_InverterState : Outport  Port=2
  hvs_EMD3_ACT_MaxAvailableTorque : Outport  Port=3
  hvs_EMD3_ACT_ReferenceTorqueLim : Outport  Port=4
  hvs_EMD3_ACT_Torque : Outport  Port=5
  hvs_EMD3_ACT_DcLinkPower : Outport  Port=6
  hvs_EMD3_ACT_MotorSpeed : Outport  Port=7
  hvs_EMD3_ACT_DcLinkVoltage : Outport  Port=8
  hvs_EMD3_ACT_MaxJunctionTemp : Outport  Port=9
  hvs_EMD3_ACT_MotorTemperature : Outport  Port=10
  hvs_EMD3_ACT_InverterLosses : Outport  Port=11
  hvs_EMD3_ACT_MotorLosses : Outport  Port=12
  wires:
  IN_EMD3_ACT_MotorLosses/1 -> hvs_EMD3_ACT_MotorLosses/1  "hvs_EMD3_ACT_MotorLosses"
  IN_EMD3_ACT_InverterLosses/1 -> hvs_EMD3_ACT_InverterLosses/1  "hvs_EMD3_ACT_InverterLosses"
  Constant5/1 -> Nm_to_percent1/2(Reference_Torque)
  IN_EMD3_ACT_ReferenceTorqueLimited/1 -> Nm_to_percent1/1(Nm_Torque)  "EMD1_ACT_ReferenceTorqueLimited"
  IN_EMD3_ACT_InverterState/1 -> hvs_EMD3_ACT_InverterState/1  "hvs_EMD3_ACT_InverterState"
  IN_EMD3_ACT_DcLinkPower/1 -> hvs_EMD3_ACT_DcLinkPower/1  "hvs_EMD3_ACT_DcLinkPower"
  IN_EMD3_ACT_DcLinkVoltage/1 -> hvs_EMD3_ACT_DcLinkVoltage/1  "hvs_EMD3_ACT_DcLinkVoltage"
  Nm_to_percent/1(Torque_Percentage) -> hvs_EMD3_ACT_MaxAvailableTorque/1  "hvs_EMD3_ACT_MaxAvailableTorque"
  Nm_to_percent1/1(Torque_Percentage) -> hvs_EMD3_ACT_ReferenceTorqueLim/1  "hvs_EMD3_ACT_ReferenceTorqueLim"
  IN_EMD3_ACT_MotorSpeed/1 -> hvs_EMD3_ACT_MotorSpeed/1  "hvs_EMD3_ACT_MotorSpeed"
  IN_EMD3_ACT_Torque/1 -> Nm_to_percent2/1(Nm_Torque)
  IN_EMD3_ACT_MaxJunctionTemperature/1 -> hvs_EMD3_ACT_MaxJunctionTemp/1  "hvs_EMD3_ACT_MaxJunctionTemp"
  IN_EMD3_ACT_MotorTemperature/1 -> hvs_EMD3_ACT_MotorTemperature/1  "hvs_EMD3_ACT_MotorTemperature"
  IN_EMD3_ACT_DigitalInput1/1 -> hvs_EMD3_ACT_DigitalInput1/1  "hvs_EMD3_ACT_DigitalInput1"
  IN_EMD3_ACT_MaximumAvailableTorque/1 -> Nm_to_percent/1(Nm_Torque)  "EMD1_ACT_MaximumAvailableTorque"
  Constant3/1 -> Nm_to_percent/2(Reference_Torque)
  Nm_to_percent2/1(Torque_Percentage) -> hvs_EMD3_ACT_Torque/1  "hvs_EMD3_ACT_Torque"
  Constant39/1 -> Nm_to_percent2/2(Reference_Torque)

== system Energy_converter_Electrical_to_Mechanical/AWR_DriveEmot/AWR 4 TX ==
  IN_EMD4_ACT_DcLinkVoltage : Inport
  IN_EMD4_ACT_DigitalInput1 : Inport  Port=2
  IN_EMD4_ACT_MaximumAvailableTorque : Inport  Port=3
  IN_EMD4_ACT_DcLinkPower : Inport  Port=4
  IN_EMD4_ACT_MotorSpeed : Inport  Port=5
  IN_EMD4_ACT_Torque : Inport  Port=6
  IN_EMD4_ACT_InverterState : Inport  Port=7
  IN_EMD4_ACT_ReferenceTorqueLimited : Inport  Port=8
  IN_EMD4_ACT_MaxJunctionTemperature : Inport  Port=9
  IN_EMD4_ACT_MotorTemperature : Inport  Port=10
  IN_EMD4_ACT_InverterLosses : Inport  Port=11
  IN_EMD4_ACT_MotorLosses : Inport  Port=12
  Constant3 : Constant  Value=RefTqeMOT
  Constant39 : Constant  Value=RefTqeMOT
  Constant5 : Constant  Value=RefTqeMOT
  Nm_to_percent : Subsystem
  Nm_to_percent1 : Subsystem
  Nm_to_percent2 : Subsystem
  hvs_EMD4_ACT_DigitalInput1 : Outport
  hvs_EMD4_ACT_InverterState : Outport  Port=2
  hvs_EMD4_ACT_MaxAvailableTorque : Outport  Port=3
  hvs_EMD4_ACT_ReferenceTorqueLim : Outport  Port=4
  hvs_EMD4_ACT_Torque : Outport  Port=5
  hvs_EMD4_ACT_DcLinkPower : Outport  Port=6
  hvs_EMD4_ACT_MotorSpeed : Outport  Port=7
  hvs_EMD4_ACT_DcLinkVoltage : Outport  Port=8
  hvs_EMD4_ACT_MaxJunctionTemperature : Outport  Port=9
  hvs_EMD4_ACT_MotorTemperature : Outport  Port=10
  hvs_EMD4_ACT_InverterLosses : Outport  Port=11
  hvs_EMD4_ACT_MotorLosses : Outport  Port=12
  wires:
  IN_EMD4_ACT_MotorLosses/1 -> hvs_EMD4_ACT_MotorLosses/1  "hvs_EMD4_ACT_MotorLosses"
  IN_EMD4_ACT_InverterLosses/1 -> hvs_EMD4_ACT_InverterLosses/1  "hvs_EMD4_ACT_InverterLosses"
  Nm_to_percent2/1(Torque_Percentage) -> hvs_EMD4_ACT_Torque/1  "hvs_EMD4_ACT_Torque"
  Constant39/1 -> Nm_to_percent2/2(Reference_Torque)
  Constant3/1 -> Nm_to_percent/2(Reference_Torque)
  IN_EMD4_ACT_MaximumAvailableTorque/1 -> Nm_to_percent/1(Nm_Torque)  "EMD2_ACT_MaximumAvailableTorque"
  IN_EMD4_ACT_DigitalInput1/1 -> hvs_EMD4_ACT_DigitalInput1/1  "hvs_EMD4_ACT_DigitalInput1"
  Nm_to_percent1/1(Torque_Percentage) -> hvs_EMD4_ACT_ReferenceTorqueLim/1  "hvs_EMD4_ACT_ReferenceTorqueLim"
  IN_EMD4_ACT_MotorTemperature/1 -> hvs_EMD4_ACT_MotorTemperature/1  "hvs_EMD4_ACT_MotorTemperature"
  IN_EMD4_ACT_MaxJunctionTemperature/1 -> hvs_EMD4_ACT_MaxJunctionTemperature/1  "hvs_EMD4_ACT_MaxJunctionTemperature"
  IN_EMD4_ACT_Torque/1 -> Nm_to_percent2/1(Nm_Torque)
  IN_EMD4_ACT_MotorSpeed/1 -> hvs_EMD4_ACT_MotorSpeed/1  "hvs_EMD4_ACT_MotorSpeed"
  Nm_to_percent/1(Torque_Percentage) -> hvs_EMD4_ACT_MaxAvailableTorque/1  "hvs_EMD4_ACT_MaxAvailableTorque"
  IN_EMD4_ACT_DcLinkVoltage/1 -> hvs_EMD4_ACT_DcLinkVoltage/1  "hvs_EMD4_ACT_DcLinkVoltage"
  IN_EMD4_ACT_DcLinkPower/1 -> hvs_EMD4_ACT_DcLinkPower/1  "hvs_EMD4_ACT_DcLinkPower"
  IN_EMD4_ACT_InverterState/1 -> hvs_EMD4_ACT_InverterState/1  "hvs_EMD4_ACT_InverterState"
  IN_EMD4_ACT_ReferenceTorqueLimited/1 -> Nm_to_percent1/1(Nm_Torque)  "EMD4_ACT_ReferenceTorqueLimited"
  Constant5/1 -> Nm_to_percent1/2(Reference_Torque)

== system Energy_converter_Electrical_to_Mechanical/AWR_DriveEmot/AWR1_4 ==
  EMD1_CMD_Commamd : Inport
  EMD1_CMD_MotorControlMode : Inport  Port=2
  EMD1_CMD_SpeedRefLim : Inport  Port=3
  EMD1_CMD_TorqueRefLim : Inport  Port=4
  HVFreigabeHW_SiRelay_D : Inport  Port=5
  vltZkBmsPhy : Inport  Port=6
  trqEmot1Phy : Inport  Port=7
  trqEmot4Phy : Inport  Port=8
  pwEmot1Phy : Inport  Port=9
  pwEmot4Phy : Inport  Port=10
  trqEmot1Max : Inport  Port=11
  trqEmot4Max : Inport  Port=12
  hvs_emot_Emot1_angVel : Inport  Port=13
  EMD4_CMD_Commamd : Inport  Port=14
  EMD4_CMD_MotorControlMode : Inport  Port=15
  EMD4_CMD_SpeedRefLim : Inport  Port=16
  EMD4_CMD_TorqueRefLim : Inport  Port=17
  HVFreigabeHW4_SiRelay_D : Inport  Port=18
  EDCU_Dig_SafetyCutOffDG1 : Inport  Port=19
  Emot1_Selection : Inport  Port=20
  Emot4_Selection : Inport  Port=21
  hvs_emot_Emot4_angVel : Inport  Port=22
  Bus Creator3 : BusCreator  Inputs=11
  Bus Creator4 : BusCreator  Inputs=2
  Bus Creator5 : BusCreator  Inputs=11
  Gain : Gain
  Gain1 : Gain
  Switch1 : Switch  Threshold=0.5
  Switch2 : Switch  Threshold=0.5
  ZeroWhenNotReady1 : Subsystem  TreatAsAtomicUnit=on
  ZeroWhenNotReady2 : Subsystem  TreatAsAtomicUnit=on
  awr1 : Electrical_converter/awr  SystemSampleTime=-1
  awr4 : Electrical_converter/awr  SystemSampleTime=-1
  awr1_4B : Outport
  wires:
  Emot1_Selection/1 -> awr1/Enable
  Emot4_Selection/1 -> awr4/Enable
  [EDCU_Dig_SafetyCutOffDG1] -> awr4/11
  EDCU_Dig_SafetyCutOffDG1/1 -> awr1/11, [EDCU_Dig_SafetyCutOffDG1]
  [vltZkBmsPhy] -> awr4/6
  EMD1_CMD_Commamd/1 -> awr1/1
  Bus Creator5/1 -> Switch2/1
  awr1/12 -> Switch2/2
  awr1/2 -> Bus Creator5/2
  awr1/3 -> Bus Creator5/3
  awr1/1 -> Gain/1
  awr1/4 -> Bus Creator5/4
  awr1/5 -> Bus Creator5/5
  awr1/8 -> Bus Creator5/8
  awr1/11 -> Bus Creator5/11
  awr1/10 -> Bus Creator5/10
  awr1/6 -> Bus Creator5/6
  awr1/7 -> Bus Creator5/7
  awr1/9 -> Bus Creator5/9
  awr4/12 -> Switch1/2
  Switch2/1 -> Bus Creator4/1  "awr1B"
  ZeroWhenNotReady1/1(Out1) -> Switch2/3
  awr4/4 -> Bus Creator3/4
  awr4/1 -> Gain1/1
  awr4/6 -> Bus Creator3/6
  awr4/7 -> Bus Creator3/7
  awr4/8 -> Bus Creator3/8
  awr4/9 -> Bus Creator3/9
  awr4/5 -> Bus Creator3/5
  awr4/11 -> Bus Creator3/11
  awr4/10 -> Bus Creator3/10
  awr4/3 -> Bus Creator3/3
  awr4/2 -> Bus Creator3/2
  Switch1/1 -> Bus Creator4/2  "awr4B"
  ZeroWhenNotReady2/1(Out1) -> Switch1/3
  Bus Creator3/1 -> Switch1/1  "awr4B"
  trqEmot1Max/1 -> awr1/9
  pwEmot1Phy/1 -> awr1/8
  trqEmot1Phy/1 -> awr1/7
  trqEmot4Max/1 -> awr4/9
  pwEmot4Phy/1 -> awr4/8
  trqEmot4Phy/1 -> awr4/7
  Bus Creator4/1 -> awr1_4B/1  "awr1_4B"
  EMD4_CMD_TorqueRefLim/1 -> awr4/4
  EMD4_CMD_Commamd/1 -> awr4/1
  EMD4_CMD_SpeedRefLim/1 -> awr4/3
  HVFreigabeHW4_SiRelay_D/1 -> awr4/5
  HVFreigabeHW_SiRelay_D/1 -> awr1/5
  EMD1_CMD_TorqueRefLim/1 -> awr1/4
  EMD1_CMD_SpeedRefLim/1 -> awr1/3
  Gain/1 -> Bus Creator5/1  "EMD1_ACT_DcLinkVoltage"
  Gain1/1 -> Bus Creator3/1  "EMD4_ACT_DcLinkVoltage"
  hvs_emot_Emot4_angVel/1 -> awr4/10
  EMD4_CMD_MotorControlMode/1 -> awr4/2
  EMD1_CMD_MotorControlMode/1 -> awr1/2
  vltZkBmsPhy/1 -> awr1/6, [vltZkBmsPhy]
  hvs_emot_Emot1_angVel/1 -> awr1/10

== system Energy_converter_Electrical_to_Mechanical/AWR_DriveEmot/AWR2_3 ==
  EMD2_CMD_Commamd : Inport
  EMD2_CMD_MotorControlMode : Inport  Port=2
  EMD2_CMD_SpeedRefLim : Inport  Port=3
  EMD2_CMD_TorqueRefLim : Inport  Port=4
  HVFreigabeHW2_SiRelay_D : Inport  Port=5
  vltZkBmsPhy : Inport  Port=6
  trqEmot2Phy : Inport  Port=7
  trqEmot3Phy : Inport  Port=8
  pwEmot2Phy : Inport  Port=9
  pwEmot3Phy : Inport  Port=10
  trqEmot2Max : Inport  Port=11
  trqEmot3Max : Inport  Port=12
  hvs_emot_Emot2_angVel : Inport  Port=13
  EMD3_CMD_Commamd : Inport  Port=14
  EMD3_CMD_MotorControlMode : Inport  Port=15
  EMD3_CMD_SpeedRefLim : Inport  Port=16
  EMD3_CMD_TorqueRefLim : Inport  Port=17
  HVFreigabeHW3_SiRelay_D : Inport  Port=18
  EDCU_Dig_SafetyCutOffDG1 : Inport  Port=19
  Emot2_Selection : Inport  Port=20
  Emot3_Selection : Inport  Port=21
  hvs_emot_Emot3_angVel : Inport  Port=22
  Bus Creator3 : BusCreator  Inputs=11
  Bus Creator4 : BusCreator  Inputs=2
  Bus Creator5 : BusCreator  Inputs=11
  Gain : Gain
  Gain1 : Gain
  Switch1 : Switch  Threshold=0.5
  Switch2 : Switch  Threshold=0.5
  ZeroWhenNotReady1 : Subsystem  TreatAsAtomicUnit=on
  ZeroWhenNotReady2 : Subsystem  TreatAsAtomicUnit=on
  awr2 : Electrical_converter/awr  SystemSampleTime=-1
  awr3 : Electrical_converter/awr  SystemSampleTime=-1
  awr2_3B : Outport
  wires:
  Emot3_Selection/1 -> awr3/Enable
  Emot2_Selection/1 -> awr2/Enable
  [EDCU_Dig_SafetyCutOffDG1] -> awr3/11
  EDCU_Dig_SafetyCutOffDG1/1 -> awr2/11, [EDCU_Dig_SafetyCutOffDG1]
  hvs_emot_Emot2_angVel/1 -> awr2/10
  vltZkBmsPhy/1 -> [vltZkBmsPhy], awr2/6
  EMD2_CMD_MotorControlMode/1 -> awr2/2
  EMD3_CMD_MotorControlMode/1 -> awr3/2
  hvs_emot_Emot3_angVel/1 -> awr3/10
  Gain1/1 -> Bus Creator3/1  "EMD3_ACT_DcLinkVoltage"
  Gain/1 -> Bus Creator5/1  "EMD2_ACT_DcLinkVoltage"
  EMD2_CMD_SpeedRefLim/1 -> awr2/3
  EMD2_CMD_TorqueRefLim/1 -> awr2/4
  HVFreigabeHW2_SiRelay_D/1 -> awr2/5
  HVFreigabeHW3_SiRelay_D/1 -> awr3/5
  EMD3_CMD_SpeedRefLim/1 -> awr3/3
  EMD3_CMD_Commamd/1 -> awr3/1
  EMD3_CMD_TorqueRefLim/1 -> awr3/4
  Bus Creator4/1 -> awr2_3B/1  "awr2_3B"
  trqEmot3Phy/1 -> awr3/7
  pwEmot3Phy/1 -> awr3/8
  trqEmot3Max/1 -> awr3/9
  trqEmot2Phy/1 -> awr2/7
  pwEmot2Phy/1 -> awr2/8
  trqEmot2Max/1 -> awr2/9
  Bus Creator3/1 -> Switch1/1  "awr4B"
  ZeroWhenNotReady2/1(Out1) -> Switch1/3
  Switch1/1 -> Bus Creator4/2  "awr3B"
  awr3/2 -> Bus Creator3/2
  awr3/3 -> Bus Creator3/3
  awr3/10 -> Bus Creator3/10
  awr3/11 -> Bus Creator3/11
  awr3/5 -> Bus Creator3/5
  awr3/9 -> Bus Creator3/9
  awr3/8 -> Bus Creator3/8
  awr3/7 -> Bus Creator3/7
  awr3/6 -> Bus Creator3/6
  awr3/1 -> Gain1/1
  awr3/4 -> Bus Creator3/4
  ZeroWhenNotReady1/1(Out1) -> Switch2/3
  Switch2/1 -> Bus Creator4/1  "awr2B"
  awr3/12 -> Switch1/2
  awr2/9 -> Bus Creator5/9
  awr2/7 -> Bus Creator5/7
  awr2/6 -> Bus Creator5/6
  awr2/10 -> Bus Creator5/10
  awr2/11 -> Bus Creator5/11
  awr2/8 -> Bus Creator5/8
  awr2/5 -> Bus Creator5/5
  awr2/4 -> Bus Creator5/4
  awr2/1 -> Gain/1
  awr2/3 -> Bus Creator5/3
  awr2/2 -> Bus Creator5/2
  awr2/12 -> Switch2/2
  Bus Creator5/1 -> Switch2/1
  EMD2_CMD_Commamd/1 -> awr2/1
  [vltZkBmsPhy] -> awr3/6

== system Energy_converter_Electrical_to_Mechanical/AWR_DriveEmot/EMD1_CMD_Command ==
  EMD1_CMD_ClearErrors : Inport
  EMD1_CMD_MotorControlMode : Inport  Port=2
  Compare To Constant : Subsystem  mask(Compare To Constant){relop===, const=1, OutDataTypeStr=boolean, ZeroCross=on}
      mask prompts: relop "Simulink:masks:Operator_MP"; const "Simulink:masks:ConstantValue_MP"; OutDataTypeStr "Simulink:masks:OutputDataType_MP"; ZeroCross "Simulink:masks:EnableZerocrossingDetection_MP"
      mask help: Simulink:masks:CompareToConstant_MD
      mask init:
      | blkName = gcb;
      | 
      | if strcmp(get_param(gcbh,'OutDataTypeStr'),'boolean')
      | 	setValue = 'boolean';
      | else
      | 	setValue = 'fixdt(0, 8)';
      | end
      | 
      | set_param([blkName,'/Compare'],'relop',relop, ...
      | 	'OutDataTypeStr', setValue, 'ZeroCross', ZeroCross);
      | 
      | str = [relop,' C']; %default
      | 
      | const_str = get_param(blkName, 'const');
      | 
      | if isempty(strfind(const_str, ' ')) && isempty(strfind(const_str, ','))
      |     % scalar or single expression
      |     if isempty(str2num(const_str))
      |         %expression
      |         str = [relop, ' ', const_str];
      |     elseif length(const) == 1
      |         str = [relop,' ',num2str(double(const))];
      |     end
      | end
      mask TypeOptions relop: == | ~= | < | <= | >= | >
      mask TypeOptions OutDataTypeStr: Simulink:masks:uint8 | Simulink:masks:boolean
      mask Callback ZeroCross: sl('zeroCrossEnable', gcbh);
      mask Display: disp(str)
  Compare To Constant1 : Subsystem  mask(Compare To Constant){relop===, const=1, OutDataTypeStr=boolean, ZeroCross=on}
      mask prompts: relop "Simulink:masks:Operator_MP"; const "Simulink:masks:ConstantValue_MP"; OutDataTypeStr "Simulink:masks:OutputDataType_MP"; ZeroCross "Simulink:masks:EnableZerocrossingDetection_MP"
      mask help: Simulink:masks:CompareToConstant_MD
      mask init: same as Energy_converter_Electrical_to_Mechanical/AWR_DriveEmot/EMD1_CMD_Command/Compare To Constant
      mask TypeOptions relop: == | ~= | < | <= | >= | >
      mask TypeOptions OutDataTypeStr: Simulink:masks:uint8 | Simulink:masks:boolean
      mask Callback ZeroCross: sl('zeroCrossEnable', gcbh);
      mask Display: disp(str)
  Constant : Constant  Value=4
  Constant3 : Constant
  Constant4 : Constant  Value=0
  Switch : Switch  Threshold=0.5
  Switch1 : Switch  Threshold=0.5
  Out_EMD1_CMD_Command : Outport
  wires:
  EMD1_CMD_MotorControlMode/1 -> Compare To Constant/1(u)
  EMD1_CMD_ClearErrors/1 -> Compare To Constant1/1(u)
  Compare To Constant1/1(y) -> Switch/2
  Switch1/1 -> Switch/3
  Constant/1 -> Switch/1
  Constant3/1 -> Switch1/1
  Constant4/1 -> Switch1/3
  Switch/1 -> Out_EMD1_CMD_Command/1
  Compare To Constant/1(y) -> Switch1/2

== system Energy_converter_Electrical_to_Mechanical/AWR_DriveEmot/EMD1_CMD_Command1 ==
  EMD1_CMD_ClearErrors : Inport
  EMD1_CMD_MotorControlMode : Inport  Port=2
  Compare To Constant : Subsystem  mask(Compare To Constant){relop===, const=1, OutDataTypeStr=boolean, ZeroCross=on}
      mask prompts: relop "Simulink:masks:Operator_MP"; const "Simulink:masks:ConstantValue_MP"; OutDataTypeStr "Simulink:masks:OutputDataType_MP"; ZeroCross "Simulink:masks:EnableZerocrossingDetection_MP"
      mask help: Simulink:masks:CompareToConstant_MD
      mask init: same as Energy_converter_Electrical_to_Mechanical/AWR_DriveEmot/EMD1_CMD_Command/Compare To Constant
      mask TypeOptions relop: == | ~= | < | <= | >= | >
      mask TypeOptions OutDataTypeStr: Simulink:masks:uint8 | Simulink:masks:boolean
      mask Callback ZeroCross: sl('zeroCrossEnable', gcbh);
      mask Display: disp(str)
  Compare To Constant1 : Subsystem  mask(Compare To Constant){relop===, const=1, OutDataTypeStr=boolean, ZeroCross=on}
      mask prompts: relop "Simulink:masks:Operator_MP"; const "Simulink:masks:ConstantValue_MP"; OutDataTypeStr "Simulink:masks:OutputDataType_MP"; ZeroCross "Simulink:masks:EnableZerocrossingDetection_MP"
      mask help: Simulink:masks:CompareToConstant_MD
      mask init: same as Energy_converter_Electrical_to_Mechanical/AWR_DriveEmot/EMD1_CMD_Command/Compare To Constant
      mask TypeOptions relop: == | ~= | < | <= | >= | >
      mask TypeOptions OutDataTypeStr: Simulink:masks:uint8 | Simulink:masks:boolean
      mask Callback ZeroCross: sl('zeroCrossEnable', gcbh);
      mask Display: disp(str)
  Constant : Constant  Value=4
  Constant3 : Constant
  Constant4 : Constant  Value=0
  Switch : Switch  Threshold=0.5
  Switch1 : Switch  Threshold=0.5
  Out_EMD1_CMD_Command : Outport
  wires:
  EMD1_CMD_MotorControlMode/1 -> Compare To Constant/1(u)
  EMD1_CMD_ClearErrors/1 -> Compare To Constant1/1(u)
  Compare To Constant1/1(y) -> Switch/2
  Switch1/1 -> Switch/3
  Constant/1 -> Switch/1
  Constant3/1 -> Switch1/1
  Constant4/1 -> Switch1/3
  Switch/1 -> Out_EMD1_CMD_Command/1
  Compare To Constant/1(y) -> Switch1/2
